simulink model "PIDSeperate"  (R2020a)
settings: Solver=VariableStepAuto  StartTime=0.0  StopTime=10.0  RelTol=1e-3
settings Model: Creator=Pranshu  LastModifiedBy=Pranshu

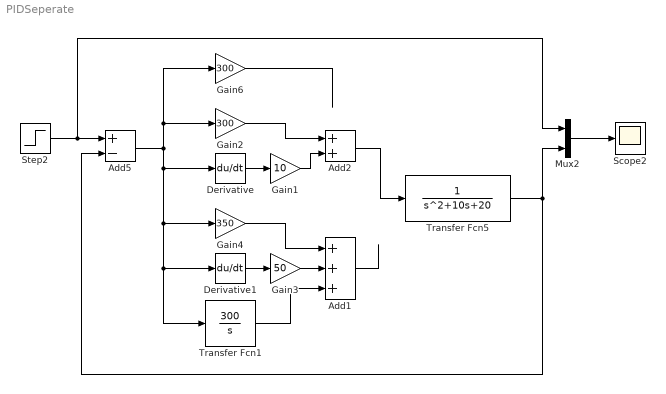
== system PIDSeperate ==
  Add1 : Sum  Inputs=+++
  Add2 : Sum
  Add5 : Sum  Inputs=+-
  Derivative : Derivative
  Derivative1 : Derivative
  Gain1 : Gain  Gain=10
  Gain2 : Gain  Gain=300
  Gain3 : Gain  Gain=50
  Gain4 : Gain  Gain=350
  Gain6 : Gain  Gain=300
  Mux2 : Mux  Inputs=2
  Scope2 : Scope
  Step2 : Step  SampleTime=0
  Transfer Fcn1 : TransferFcn  Numerator=[300]  Denominator=[1 0]
  Transfer Fcn5 : TransferFcn  Denominator=[1 10 20]
  wires:
  Mux2/1 -> Scope2/1
  Step2/1 -> Add5/1, Mux2/1
  Transfer Fcn5/1 -> Mux2/2, Add5/2
  Gain6/1 -> ?
  Derivative/1 -> Gain1/1
  Add2/1 -> Transfer Fcn5/1
  Gain1/1 -> Add2/2
  Gain2/1 -> Add2/1
  Gain4/1 -> Add1/1
  Add5/1 -> Gain2/1, Gain6/1, Gain4/1, Transfer Fcn1/1, Derivative1/1, Derivative/1
  Gain3/1 -> Add1/2
  Derivative1/1 -> Gain3/1
  Transfer Fcn1/1 -> Add1/3
  Add1/1 -> ?
